simulink model "stepdowncycloconverter_2_final_gto"  (R2022b)
settings: Solver=VariableStepAuto  StartTime=0.0  StopTime=20  MaxStep=0.0001  RelTol=1e-3
libraries: spsGtoLib x8, spsVoltageMeasurementLib x2, spsACVoltageSourceLib x1, spsSeriesRLCBranchLib x1, sps_lib x1
settings Model: Creator=hp  LastModifiedBy=hp

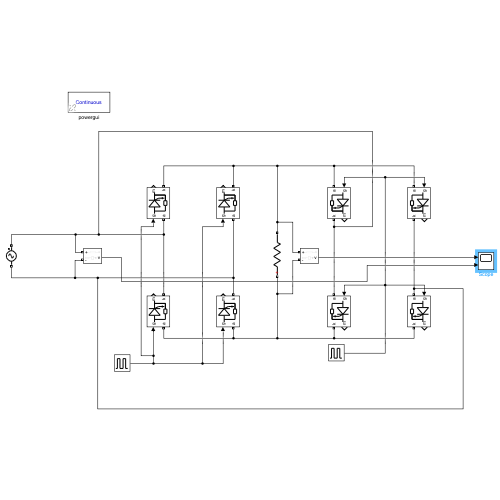
[thumbnail: Simulink's stored preview of the top-level diagram]
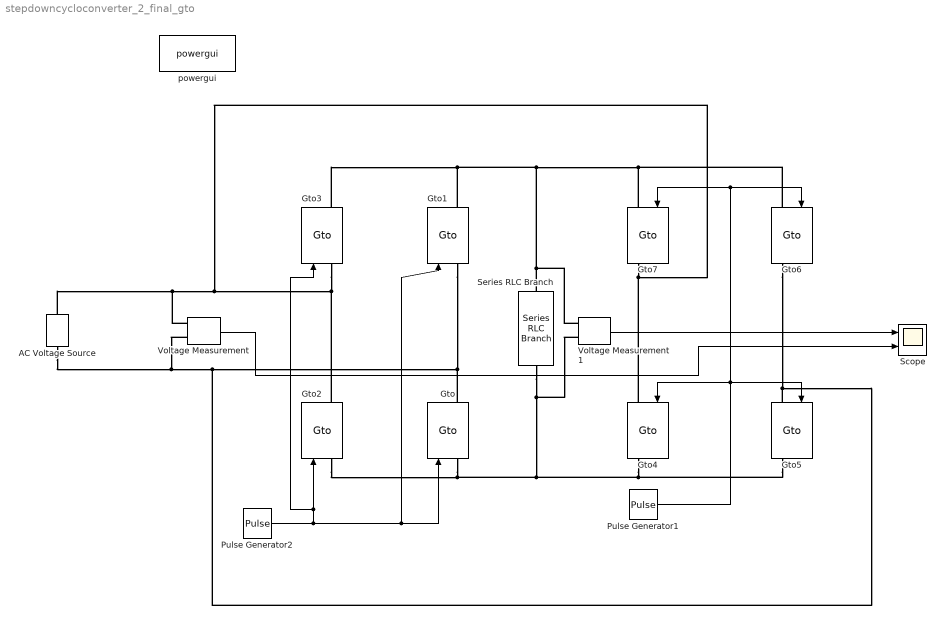
== system stepdowncycloconverter_2_final_gto ==
  AC Voltage Source : spsACVoltageSourceLib/AC Voltage Source  Amplitude=230  Phase=0  Frequency=50  SampleTime=0  Measurements=None  BusType=swing  Pref=10e3  Qref=0  Qmin=-inf  Qmax=+inf
  Gto{,1..7} (8 alike) : spsGtoLib/Gto  Ron=0.001  Lon=0  Vf=1  Tf=10e-6  Tt=20e-6  IC=0  Rs=1e5  Cs=inf  Measurements=on
      settings: LibrarySourceBlock=sps_lib/Power Electronics/Gto
  Pulse Generator1 : DiscretePulseGenerator  PulseType=Time based  Period=0.08  PulseWidth=50  PhaseDelay=0.04
  Pulse Generator2 : DiscretePulseGenerator  PulseType=Time based  Period=0.08  PulseWidth=50
  Scope : Scope  NumInputPorts=2
  Series RLC Branch : spsSeriesRLCBranchLib/Series RLC Branch  LConnTagsString=__new0  RConnTagsString=__new0  BranchType=R  Resistance=1  Inductance=1e-3  SetiL0=off  InitialCurrent=0  Capacitance=1e-6  Setx0=off  InitialVoltage=0  Measurements=None
  Voltage Measurement : spsVoltageMeasurementLib/Voltage Measurement  PhasorSimulation=off  OutputType=Complex  PSBequivalent=0
  Voltage Measurement1 : spsVoltageMeasurementLib/Voltage Measurement  PhasorSimulation=off  OutputType=Complex  PSBequivalent=0
  powergui : sps_lib/powergui  Priority=1  SimulationMode=Continuous  SampleTime=50e-6  frequency=50  Iterations=50  frequencyindice=50  Pbase=100e6  ErrMax=1e-4  UnitsV=kV  UnitsW=MW  buscounter=0  FunctionMessages=off  echomessages=off  EnableUseOfTLC=off  CurrentSourceSwitches=off  DisableSnubberDevices=off  DisableRonSwitches=off  DisableVfSwitches=off  DisplayEquations=off  AutomaticDiscreteSolvers=off  SolverType=Tustin/Backward Euler (TBE)  Interpol=off  ExternalGateDelay=off  methode=off  Ts=100  x0status=blocks  SPID=on  SwTol=0  HookPort=off  NonlinearTolerance=1e-4  nMaxIteration=100  ContinueOnMaxIteration=off  RestoreLinks=warning  ResistiveCurrentMeasurement=off  Frange=[0:2:500]  Ylog=off  Xlog=on  ShowGrid=off  save=off  variable=ZData  structure=0  ZoomFFT=off  StartTime=0.0  cycles=1  DisplayStyle=1  fundamental=60  FreqAxis=off  MaxFrequency=1000  frequencyindicesteady=1  RmsSteady=1  display=off
  wires:
  Voltage Measurement/1 -> Scope/2
  Pulse Generator2/1 -> Gto/1, Gto1/1, Gto2/1, Gto3/1
  Pulse Generator1/1 -> Gto4/1, Gto5/1, Gto6/1, Gto7/1
  Voltage Measurement1/1 -> Scope/1
  connections:
  AC Voltage Source/RConn1 -- Voltage Measurement/LConn1 -- Gto4/LConn1 -- Gto7/RConn1 -- Gto2/RConn1 -- Gto3/LConn1
  Voltage Measurement/LConn2 -- AC Voltage Source/LConn1 -- Gto6/RConn1 -- Gto5/LConn1 -- Gto1/LConn1 -- Gto/RConn1
  Voltage Measurement1/LConn1 -- Series RLC Branch/RConn1 -- Gto6/LConn1 -- Gto7/LConn1 -- Gto1/RConn1 -- Gto3/RConn1
  Series RLC Branch/LConn1 -- Voltage Measurement1/LConn2 -- Gto4/RConn1 -- Gto5/RConn1 -- Gto2/LConn1 -- Gto/LConn1
